simulink model "fourierseries"  (R2024b)
settings: Solver=VariableStepAuto  StartTime=0.0  StopTime=180  RelTol=1e-3
settings Model: Creator=castl  LastModifiedBy=castl

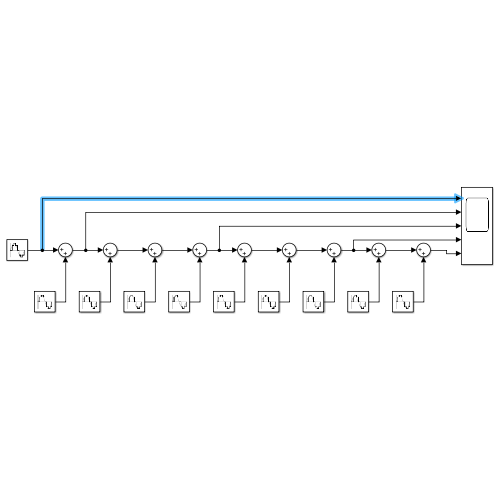
[thumbnail: Simulink's stored preview of the top-level diagram]
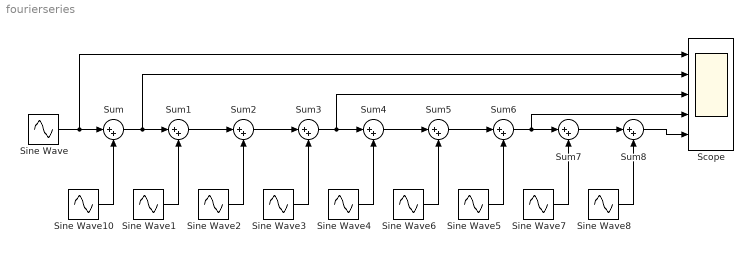
== system fourierseries ==
  Scope : Scope  NumInputPorts=5
  Sine Wave : Sin  Amplitude=4/pi  Frequency=2*pi/92  Phase=pi/2  SampleTime=0.1
  Sine Wave1 : Sin  Amplitude=4/pi*(1/5)  Frequency=5*(2*pi/92)  Phase=pi/2  SampleTime=0.1
  Sine Wave10 : Sin  Amplitude=4/pi*(-1/3)  Frequency=3*(2*pi/92)  Phase=pi/2  SampleTime=0.1
  Sine Wave2 : Sin  Amplitude=4/pi*(-1/7)  Frequency=7*(2*pi/92)  Phase=pi/2  SampleTime=0.1
  Sine Wave3 : Sin  Amplitude=4/pi*(1/9)  Frequency=9*(2*pi/92)  Phase=pi/2  SampleTime=0.1
  Sine Wave4 : Sin  Amplitude=4/pi*(-1/11)  Frequency=11*(2*pi/92)  Phase=pi/2  SampleTime=0.1
  Sine Wave5 : Sin  Amplitude=4/pi*(-1/15)  Frequency=15*(2*pi/92)  Phase=pi/2  SampleTime=0.1
  Sine Wave6 : Sin  Amplitude=4/pi*(1/13)  Frequency=13*(2*pi/92)  Phase=pi/2  SampleTime=0.1
  Sine Wave7 : Sin  Amplitude=4/pi*(1/17)  Frequency=17*(2*pi/92)  Phase=pi/2  SampleTime=0.1
  Sine Wave8 : Sin  Amplitude=4/pi*(-1/19)  Frequency=19*(2*pi/92)  Phase=pi/2  SampleTime=0.1
  Sum{,1..8} (9 alike) : Sum  Inputs=|++
  wires:
  Sum2/1 -> Sum3/1
  Sum4/1 -> Sum5/1
  Sum3/1 -> Scope/3, Sum4/1
  Sum1/1 -> Sum2/1
  Sum/1 -> Scope/2, Sum1/1
  Sine Wave/1 -> Scope/1, Sum/1
  Sine Wave10/1 -> Sum/2
  Sine Wave1/1 -> Sum1/2
  Sine Wave2/1 -> Sum2/2
  Sine Wave3/1 -> Sum3/2
  Sine Wave4/1 -> Sum4/2
  Sine Wave5/1 -> Sum6/2
  Sine Wave7/1 -> Sum7/2
  Sine Wave8/1 -> Sum8/2
  Sum5/1 -> Sum6/1
  Sum6/1 -> Scope/4, Sum7/1
  Sum7/1 -> Sum8/1
  Sum8/1 -> Scope/5
  Sine Wave6/1 -> Sum5/2
